simulink model "modele_detaille_LIMA_MILITAO_PINHEIRO"  (R2019a)
settings: Solver=ode45  StartTime=0.0  StopTime=8  RelTol=1e-4  EnableMultiTasking=on
undefined symbols (not defined in the file): fa, fm, G1, G_den_RST, G_num_RST, Ja, Jm, Jt, ka, kt, R, R1, ro, S, T, Te, tsim
settings Model: Creator=xshi  LastModifiedBy=dougl
settings DataIOCC: LimitDataPoints=on  SaveFormat=Array  SignalLoggingSaveFormat=ModelDataLogs  ReturnWorkspaceOutputs=off  SignalLoggingName=sigsOut
settings DebuggingCC: SaveWithParameterizedLinksMsg=none  UnderspecifiedInitializationDetection=Classic  MergeDetectMultiDrivingBlocksExec=none  SignalResolutionControl=TryResolveAllWithWarning  MultiTaskDSMMsg=warning  MultiTaskCondExecSysMsg=none
settings HardwareCC: ProdBitPerPointer=32  ProdBitPerSizeT=32  ProdBitPerPtrDiffT=32  ProdLargestAtomicFloat=None  ProdIntDivRoundTo=Undefined  ProdEndianess=Unspecified  ProdWordSize=32  ProdHWDeviceType=32-bit Generic  TargetUnknown=on
settings ModelReferenceCC: PropagateSignalLabelsOutOfModel=off
settings GRTTargetCC: CombineOutputUpdateFcns=off  GRTInterface=on
settings ConfigComp: CovMetricSettings=dw  CovSaveCumulativeToWorkspaceVar=on  CovSaveSingleToWorkspaceVar=on

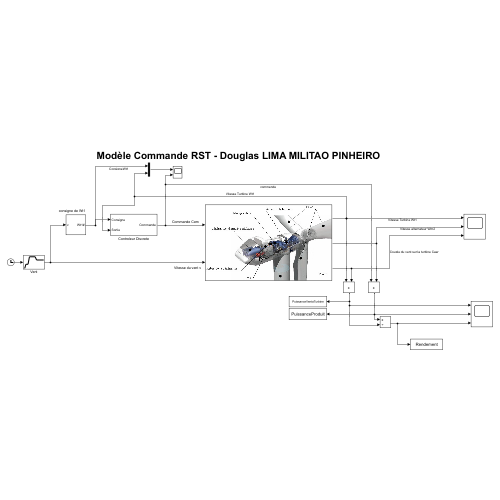
[thumbnail: Simulink's stored preview of the top-level diagram]
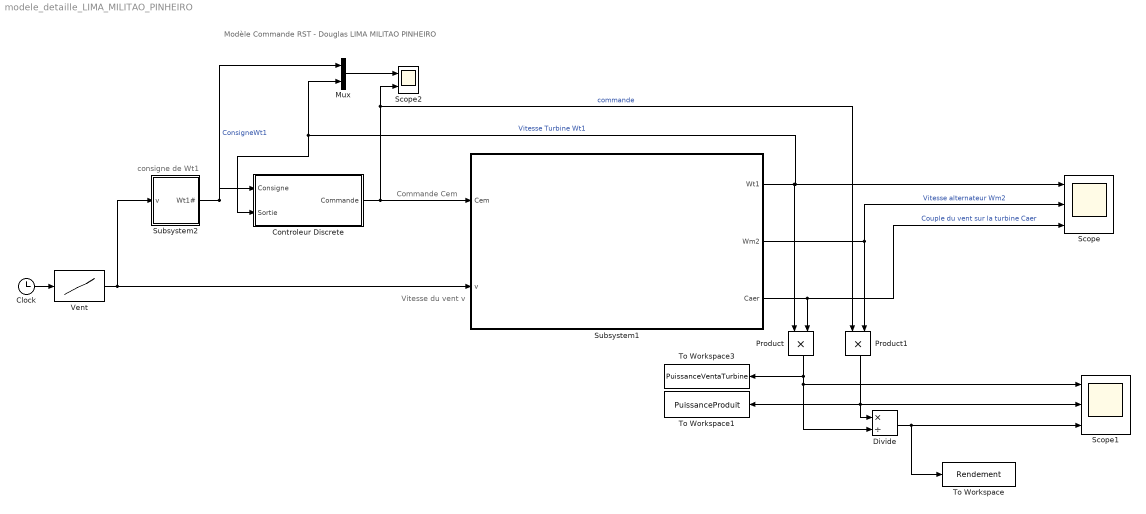
== system modele_detaille_LIMA_MILITAO_PINHEIRO ==
  note: consigne de Wt1
  note: Vitesse du vent v
  note: Commande Cem
  note: Modèle Commande RST - Douglas LIMA MILITAO PINHEIRO
  Clock : Clock
  Controleur Discrete : Subsystem
  Divide : Product  Inputs=*/
  Mux : Mux  Inputs=2
  Product : Product
  Product1 : Product
  Scope : Scope  NumInputPorts=3
  Scope1 : Scope  NumInputPorts=3
  Scope2 : Scope  NumInputPorts=2
  Subsystem1 : Subsystem
      mask Display:
      | image('eolienne.jpg');
      | %port_label('output', 1, 'référence vitesse turbine');
      | %port_label('output', 2, 'vitesse turbine');
      | %port_label('output', 3, 'vitesse alternateur');
      | %port_label('input', 1, 'Vitese du vent v');
      | %port_label('input', 2, 'Commande Cem');
  Subsystem2 : Subsystem
  To Workspace : ToWorkspace  VariableName=Rendement  SampleTime=tsim
  To Workspace1 : ToWorkspace  VariableName=PuissanceProduit  SampleTime=tsim
  To Workspace3 : ToWorkspace  VariableName=PuissanceVentaTurbine  SampleTime=tsim
  Vent : Lookup  InputValues="[0 0.1 0.6 1.5 2 4.5 5  6  8]"  Table=[0 0 5 5 14 14 10 10 10]  SaturateOnIntegerOverflow=on
  wires:
  Clock/1 -> Vent/1
  Vent/1 -> Subsystem1/2(v), Subsystem2/1(v)
  Subsystem2/1(Wt1#) -> Mux/1, Controleur Discrete/1(Consigne)  "ConsigneWt1"
  Subsystem1/2(Wm2) -> Product1/2, Scope/2  "Vitesse alternateur Wm2"
  Subsystem1/3(Caer) -> Product/2, Scope/3  "Couple du vent sur la turbine Caer"
  Subsystem1/1(Wt1) -> Scope/1, Controleur Discrete/2(Sortie), Mux/2, Product/1  "Vitesse Turbine Wt1"
  Mux/1 -> Scope2/1
  Controleur Discrete/1(Commande) -> Subsystem1/1(Cem), Product1/1, Scope2/2  "commande"
  Product/1 -> Divide/2, Scope1/1, To Workspace3/1
  Product1/1 -> Divide/1, To Workspace1/1, Scope1/2
  Divide/1 -> To Workspace/1, Scope1/3

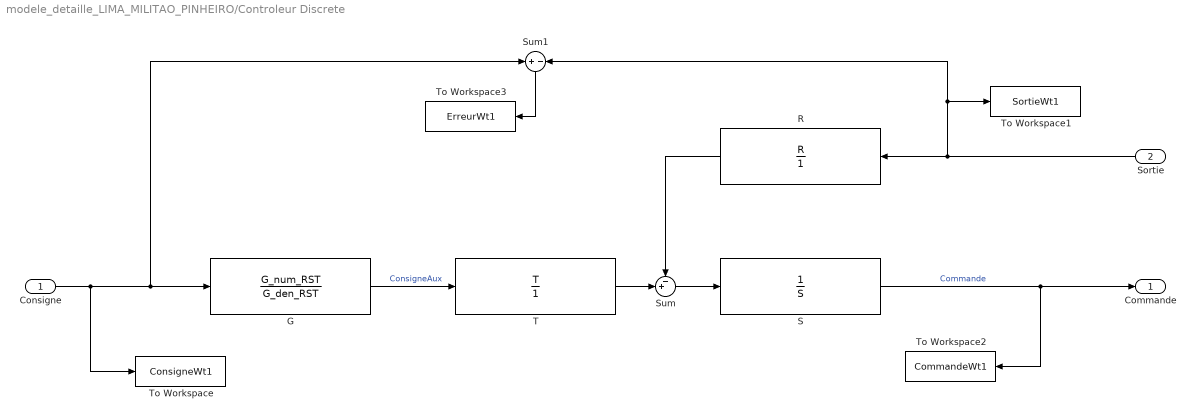
== system modele_detaille_LIMA_MILITAO_PINHEIRO/Controleur Discrete ==
  Consigne : Inport
  Sortie : Inport  Port=2
  G : DiscreteFilter  Numerator=G_num_RST  Denominator=G_den_RST  SampleTime=Te
  R : DiscreteFilter  Numerator=R  Denominator=1  SampleTime=Te
  S : DiscreteFilter  Numerator=1  Denominator=S  SampleTime=Te
  Sum : Sum  Inputs=-+|
  Sum1 : Sum  Inputs=+|-
  T : DiscreteFilter  Numerator=T  Denominator=1  SampleTime=Te
  To Workspace : ToWorkspace  VariableName=ConsigneWt1  SampleTime=tsim
  To Workspace1 : ToWorkspace  VariableName=SortieWt1  SampleTime=tsim
  To Workspace2 : ToWorkspace  VariableName=CommandeWt1  SampleTime=tsim
  To Workspace3 : ToWorkspace  VariableName=ErreurWt1  SampleTime=tsim
  Commande : Outport
  wires:
  Consigne/1 -> To Workspace/1, Sum1/1, G/1
  G/1 -> T/1  "ConsigneAux"
  T/1 -> Sum/2
  Sum/1 -> S/1
  R/1 -> Sum/1
  Sortie/1 -> Sum1/2, To Workspace1/1, R/1
  S/1 -> Commande/1, To Workspace2/1  "Commande"
  Sum1/1 -> To Workspace3/1

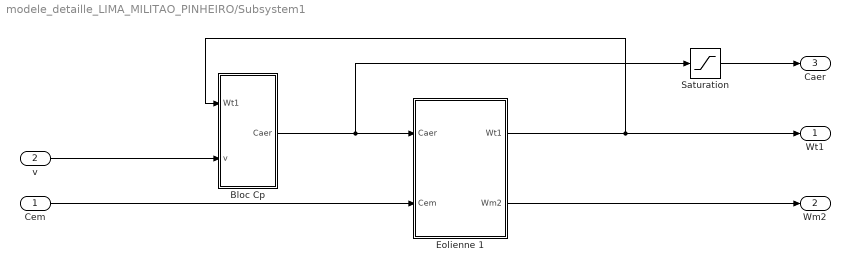
== system modele_detaille_LIMA_MILITAO_PINHEIRO/Subsystem1 ==
  Cem : Inport
  v : Inport  Port=2
  Bloc Cp : Subsystem
  Eolienne 1 : Subsystem
  Saturation : Saturate  UpperLimit=50e3  LowerLimit=-50e3
  Wt1 : Outport
  Wm2 : Outport  Port=2
  Caer : Outport  Port=3
  wires:
  Eolienne 1/1(Wt1) -> Wt1/1, Bloc Cp/1(Wt1)
  v/1 -> Bloc Cp/2(v)
  Bloc Cp/1(Caer) -> Saturation/1, Eolienne 1/1(Caer)
  Cem/1 -> Eolienne 1/2(Cem)
  Eolienne 1/2(Wm2) -> Wm2/1
  Saturation/1 -> Caer/1

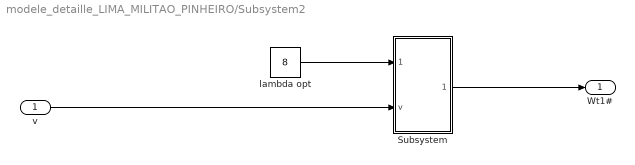
== system modele_detaille_LIMA_MILITAO_PINHEIRO/Subsystem2 ==
  v : Inport
  Subsystem : Subsystem
  lambda opt : Constant  Value=8
  Wt1# : Outport
  wires:
  lambda opt/1 -> Subsystem/1(Lambda opt)
  v/1 -> Subsystem/2(v)
  Subsystem/1(Wt1#) -> Wt1#/1

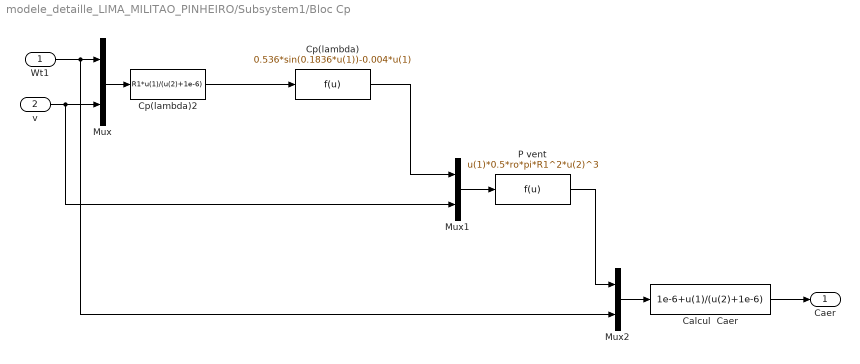
== system modele_detaille_LIMA_MILITAO_PINHEIRO/Subsystem1/Bloc Cp ==
  Wt1 : Inport
  v : Inport  Port=2
  Calcul  Caer : Fcn  Expr=1e-6+u(1)/(u(2)+1e-6)
  Cp(lambda) : Fcn  Expr=0.536*sin(0.1836*u(1))-0.004*u(1)
  Cp(lambda)2 : Fcn  Expr=R1*u(1)/(u(2)+1e-6)
  Mux : Mux  Inputs=2
  Mux1 : Mux  Inputs=2
  Mux2 : Mux  Inputs=2
  P vent : Fcn  Expr=u(1)*0.5*ro*pi*R1^2*u(2)^3
  Caer : Outport
  wires:
  Mux/1 -> Cp(lambda)2/1
  Cp(lambda)2/1 -> Cp(lambda)/1
  Wt1/1 -> Mux/1, Mux2/2
  Cp(lambda)/1 -> Mux1/1
  v/1 -> Mux/2, Mux1/2
  Mux1/1 -> P vent/1
  P vent/1 -> Mux2/1
  Mux2/1 -> Calcul  Caer/1
  Calcul  Caer/1 -> Caer/1

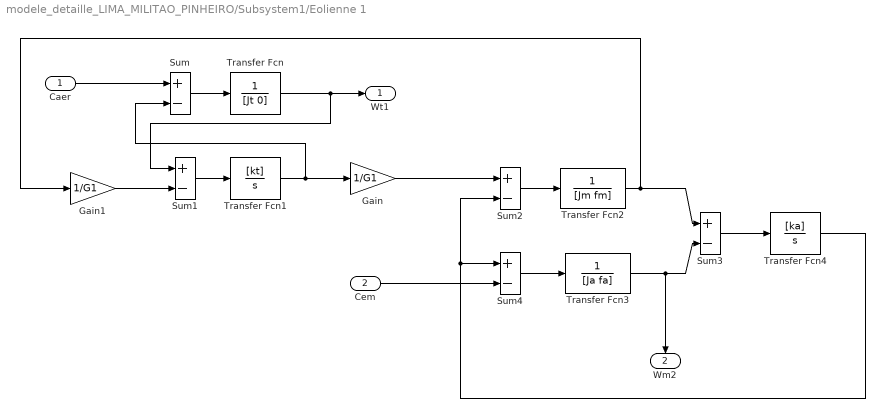
== system modele_detaille_LIMA_MILITAO_PINHEIRO/Subsystem1/Eolienne 1 ==
  Caer : Inport
  Cem : Inport  Port=2
  Gain : Gain  Gain=1/G1  SaturateOnIntegerOverflow=on  OutDataTypeStr=Inherit: Same as input  ParamDataTypeStr=Inherit: Same as input
  Gain1 : Gain  Gain=1/G1  SaturateOnIntegerOverflow=on  OutDataTypeStr=Inherit: Same as input  ParamDataTypeStr=Inherit: Same as input
  Sum{,1..4} (5 alike) : Sum  Inputs=+-  SaturateOnIntegerOverflow=on
  Transfer Fcn : TransferFcn  Denominator=[Jt 0]
  Transfer Fcn1 : TransferFcn  Numerator=[kt]  Denominator=[1 0]
  Transfer Fcn2 : TransferFcn  Denominator=[Jm fm]
  Transfer Fcn3 : TransferFcn  Denominator=[Ja fa]
  Transfer Fcn4 : TransferFcn  Numerator=[ka]  Denominator=[1 0]
  Wt1 : Outport
  Wm2 : Outport  Port=2
  wires:
  Sum/1 -> Transfer Fcn/1
  Sum1/1 -> Transfer Fcn1/1
  Transfer Fcn1/1 -> Sum/2, Gain/1
  Transfer Fcn/1 -> Sum1/1, Wt1/1
  Gain1/1 -> Sum1/2
  Gain/1 -> Sum2/1
  Sum2/1 -> Transfer Fcn2/1
  Transfer Fcn2/1 -> Sum3/1, Gain1/1
  Transfer Fcn3/1 -> Sum3/2, Wm2/1
  Sum4/1 -> Transfer Fcn3/1
  Sum3/1 -> Transfer Fcn4/1
  Transfer Fcn4/1 -> Sum2/2, Sum4/1
  Cem/1 -> Sum4/2
  Caer/1 -> Sum/1

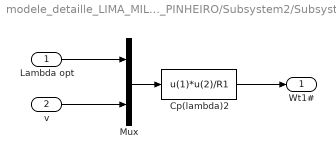
== system modele_detaille_LIMA_MILITAO_PINHEIRO/Subsystem2/Subsystem ==
  Lambda opt : Inport
  v : Inport  Port=2
  Cp(lambda)2 : Fcn  Expr=u(1)*u(2)/R1
  Mux : Mux  Inputs=2
  Wt1# : Outport
  wires:
  Mux/1 -> Cp(lambda)2/1
  v/1 -> Mux/2
  Cp(lambda)2/1 -> Wt1#/1
  Lambda opt/1 -> Mux/1
